simulink model "NonlinearPendulumSystem"  (R2014a)
settings: Solver=ode45  StartTime=0.0  StopTime=10.0  RelTol=1e-3
settings Model: Creator=User  LastModifiedBy=User

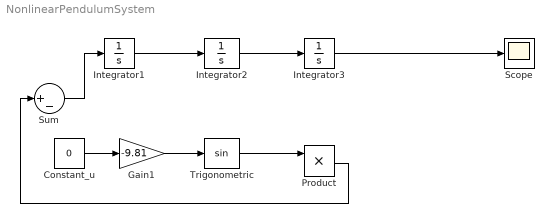
== system NonlinearPendulumSystem ==
  Constant_u : Constant  Value=0
  Gain1 : Gain  Gain=-9.81
  Integrator1 : Integrator  InitialCondition=1
  Integrator2 : Integrator
  Integrator3 : Integrator
  Product : Product
  Scope : Scope
  Sum : Sum  Inputs=|+-
  Trigonometric : Trigonometry
  wires:
  Constant_u/1 -> Gain1/1
  Gain1/1 -> Trigonometric/1
  Trigonometric/1 -> Product/1
  Product/1 -> Sum/1
  Sum/1 -> Integrator1/1
  Integrator1/1 -> Integrator2/1
  Integrator2/1 -> Integrator3/1
  Integrator3/1 -> Scope/1
